simulink model "final_heart_sym4_7_Level_double"  (R2021a)
settings: Solver=VariableStepAuto  StartTime=0.0  StopTime=8  RelTol=1e-3
undefined symbols (not defined in the file): lambda2
libraries: dspsigops x15, dspquant2 x1
(part 2 of 4)

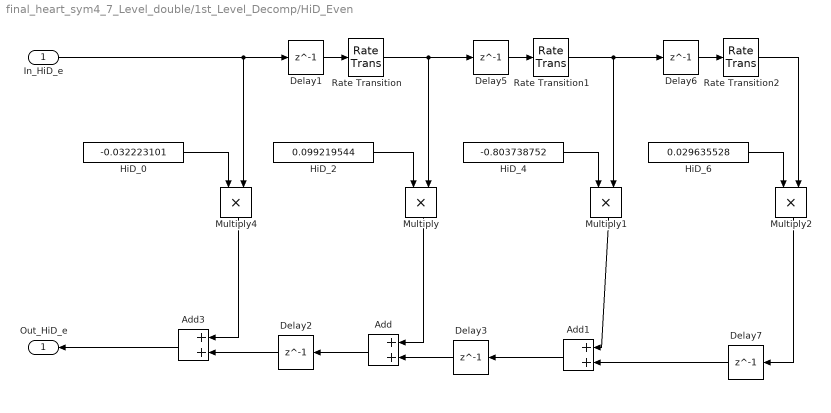
== system final_heart_sym4_7_Level_double/1st_Level_Decomp/HiD_Even ==
  In_HiD_e : Inport  OutDataTypeStr=double  SampleTime=1/44100
  Add : Sum  AccumDataTypeStr=double  OutDataTypeStr=double
  Add1 : Sum  AccumDataTypeStr=double  OutDataTypeStr=double
  Add3 : Sum  AccumDataTypeStr=double  OutDataTypeStr=double
  Delay{1..3,5..7} (6 alike) : Delay  DelayLength=1  SampleTime=1/44100
  HiD_0 : Constant  Value=-0.032223101  OutDataTypeStr=double  SampleTime=1/44100
  HiD_2 : Constant  Value=0.099219544  OutDataTypeStr=double  SampleTime=1/44100
  HiD_4 : Constant  Value=-0.803738752  OutDataTypeStr=double  SampleTime=1/44100
  HiD_6 : Constant  Value=0.029635528  OutDataTypeStr=double  SampleTime=1/44100
  Multiply{,1..2,4} (4 alike) : Product  OutDataTypeStr=double
  Rate Transition : RateTransition  OutPortSampleTime=1/44100
  Rate Transition1 : RateTransition  OutPortSampleTime=1/44100
  Rate Transition2 : RateTransition  OutPortSampleTime=1/44100
  Out_HiD_e : Outport  OutDataTypeStr=double  SampleTime=1/44100  VectorParamsAs1DForOutWhenUnconnected=off
  wires:
  Rate Transition2/1 -> Multiply2/2
  Multiply2/1 -> Delay7/1
  HiD_0/1 -> Multiply4/1
  Delay3/1 -> Add/2
  HiD_6/1 -> Multiply2/1
  In_HiD_e/1 -> Delay1/1, Multiply4/2
  HiD_2/1 -> Multiply/1
  Add3/1 -> Out_HiD_e/1
  Multiply/1 -> Add/1
  Rate Transition/1 -> Delay5/1, Multiply/2
  HiD_4/1 -> Multiply1/1
  Delay6/1 -> Rate Transition2/1
  Delay1/1 -> Rate Transition/1
  Delay7/1 -> Add1/2
  Multiply1/1 -> Add1/1
  Rate Transition1/1 -> Delay6/1, Multiply1/2
  Delay2/1 -> Add3/2
  Multiply4/1 -> Add3/1
  Delay5/1 -> Rate Transition1/1
  Add/1 -> Delay2/1
  Add1/1 -> Delay3/1

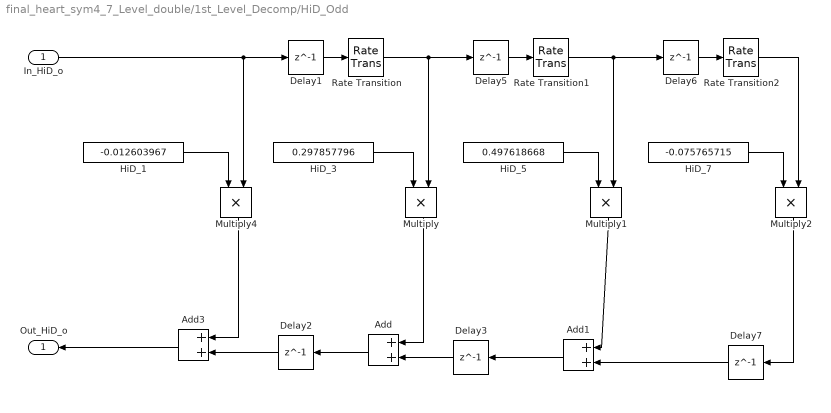
== system final_heart_sym4_7_Level_double/1st_Level_Decomp/HiD_Odd ==
  In_HiD_o : Inport  OutDataTypeStr=double  SampleTime=1/44100
  Add : Sum  AccumDataTypeStr=double  OutDataTypeStr=double
  Add1 : Sum  AccumDataTypeStr=double  OutDataTypeStr=double
  Add3 : Sum  AccumDataTypeStr=double  OutDataTypeStr=double
  Delay{1..3,5..7} (6 alike) : Delay  DelayLength=1  SampleTime=1/44100
  HiD_1 : Constant  Value=-0.012603967  OutDataTypeStr=double  SampleTime=1/44100
  HiD_3 : Constant  Value=0.297857796  OutDataTypeStr=double  SampleTime=1/44100
  HiD_5 : Constant  Value=0.497618668  OutDataTypeStr=double  SampleTime=1/44100
  HiD_7 : Constant  Value=-0.075765715  OutDataTypeStr=double  SampleTime=1/44100
  Multiply{,1..2,4} (4 alike) : Product  OutDataTypeStr=double
  Rate Transition : RateTransition  OutPortSampleTime=1/44100
  Rate Transition1 : RateTransition  OutPortSampleTime=1/44100
  Rate Transition2 : RateTransition  OutPortSampleTime=1/44100
  Out_HiD_o : Outport  OutDataTypeStr=double  SampleTime=1/44100  VectorParamsAs1DForOutWhenUnconnected=off
  wires:
  Delay1/1 -> Rate Transition/1
  Delay6/1 -> Rate Transition2/1
  Rate Transition/1 -> Delay5/1, Multiply/2
  HiD_5/1 -> Multiply1/1
  Rate Transition1/1 -> Delay6/1, Multiply1/2
  Delay2/1 -> Add3/2
  Multiply1/1 -> Add1/1
  Add1/1 -> Delay3/1
  Delay5/1 -> Rate Transition1/1
  Delay7/1 -> Add1/2
  Add/1 -> Delay2/1
  In_HiD_o/1 -> Delay1/1, Multiply4/2
  Multiply4/1 -> Add3/1
  Multiply/1 -> Add/1
  Add3/1 -> Out_HiD_o/1
  HiD_3/1 -> Multiply/1
  HiD_1/1 -> Multiply4/1
  Delay3/1 -> Add/2
  Multiply2/1 -> Delay7/1
  Rate Transition2/1 -> Multiply2/2
  HiD_7/1 -> Multiply2/1

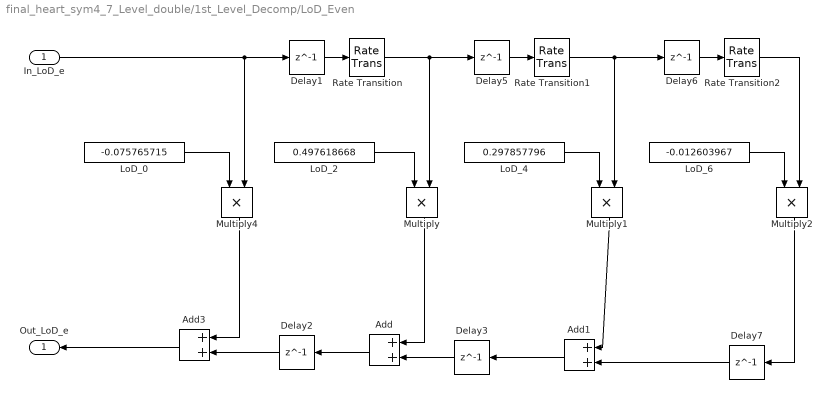
== system final_heart_sym4_7_Level_double/1st_Level_Decomp/LoD_Even ==
  In_LoD_e : Inport  OutDataTypeStr=double  SampleTime=1/44100
  Add : Sum  AccumDataTypeStr=double  OutDataTypeStr=double
  Add1 : Sum  AccumDataTypeStr=double  OutDataTypeStr=double
  Add3 : Sum  AccumDataTypeStr=double  OutDataTypeStr=double
  Delay{1..3,5..7} (6 alike) : Delay  DelayLength=1  SampleTime=1/44100
  LoD_0 : Constant  Value=-0.075765715  OutDataTypeStr=double  SampleTime=1/44100
  LoD_2 : Constant  Value=0.497618668  OutDataTypeStr=double  SampleTime=1/44100
  LoD_4 : Constant  Value=0.297857796  OutDataTypeStr=double  SampleTime=1/44100
  LoD_6 : Constant  Value=-0.012603967  OutDataTypeStr=double  SampleTime=1/44100
  Multiply{,1..2,4} (4 alike) : Product  OutDataTypeStr=double
  Rate Transition : RateTransition  OutPortSampleTime=1/44100
  Rate Transition1 : RateTransition  OutPortSampleTime=1/44100
  Rate Transition2 : RateTransition  OutPortSampleTime=1/44100
  Out_LoD_e : Outport  OutDataTypeStr=double  SampleTime=1/44100  VectorParamsAs1DForOutWhenUnconnected=off
  wires:
  Delay1/1 -> Rate Transition/1
  Delay6/1 -> Rate Transition2/1
  Rate Transition/1 -> Delay5/1, Multiply/2
  LoD_4/1 -> Multiply1/1
  Rate Transition1/1 -> Delay6/1, Multiply1/2
  Delay2/1 -> Add3/2
  Multiply1/1 -> Add1/1
  Add1/1 -> Delay3/1
  Delay5/1 -> Rate Transition1/1
  Delay7/1 -> Add1/2
  Add/1 -> Delay2/1
  In_LoD_e/1 -> Delay1/1, Multiply4/2
  Multiply4/1 -> Add3/1
  Multiply/1 -> Add/1
  Add3/1 -> Out_LoD_e/1
  LoD_2/1 -> Multiply/1
  LoD_0/1 -> Multiply4/1
  Delay3/1 -> Add/2
  Multiply2/1 -> Delay7/1
  Rate Transition2/1 -> Multiply2/2
  LoD_6/1 -> Multiply2/1

== system final_heart_sym4_7_Level_double/1st_Level_Decomp/LoD_Odd ==
  In_LoD_o : Inport  OutDataTypeStr=double  SampleTime=1/44100
  Add : Sum  AccumDataTypeStr=double  OutDataTypeStr=double
  Add1 : Sum  AccumDataTypeStr=double  OutDataTypeStr=double
  Add3 : Sum  AccumDataTypeStr=double  OutDataTypeStr=double
  Delay{1..3,5..7} (6 alike) : Delay  DelayLength=1  SampleTime=1/44100
  LoD_1 : Constant  Value=-0.029635528  OutDataTypeStr=double  SampleTime=1/44100
  LoD_3 : Constant  Value=0.803738752  OutDataTypeStr=double  SampleTime=1/44100
  LoD_5 : Constant  Value=-0.099219544  OutDataTypeStr=double  SampleTime=1/44100
  LoD_7 : Constant  Value=0.032223101  OutDataTypeStr=double  SampleTime=1/44100
  Multiply{,1..2,4} (4 alike) : Product  OutDataTypeStr=double
  Rate Transition : RateTransition  OutPortSampleTime=1/44100
  Rate Transition1 : RateTransition  OutPortSampleTime=1/44100
  Rate Transition2 : RateTransition  OutPortSampleTime=1/44100
  Out_LoD_o : Outport  OutDataTypeStr=double  SampleTime=1/44100  VectorParamsAs1DForOutWhenUnconnected=off
  wires:
  Rate Transition/1 -> Delay5/1, Multiply/2
  Add/1 -> Delay2/1
  Add1/1 -> Delay3/1
  Delay7/1 -> Add1/2
  Delay5/1 -> Rate Transition1/1
  Rate Transition1/1 -> Delay6/1, Multiply1/2
  Delay2/1 -> Add3/2
  LoD_5/1 -> Multiply1/1
  Rate Transition2/1 -> Multiply2/2
  LoD_7/1 -> Multiply2/1
  Multiply2/1 -> Delay7/1
  Delay3/1 -> Add/2
  LoD_3/1 -> Multiply/1
  Add3/1 -> Out_LoD_o/1
  Multiply/1 -> Add/1
  Multiply4/1 -> Add3/1
  Multiply1/1 -> Add1/1
  Delay6/1 -> Rate Transition2/1
  In_LoD_o/1 -> Delay1/1, Multiply4/2
  LoD_1/1 -> Multiply4/1
  Delay1/1 -> Rate Transition/1

== system final_heart_sym4_7_Level_double/1st_Level_Recon/HiR_Even ==
  In_HiR_e : Inport  OutDataTypeStr=double  SampleTime=1/44100
  Add1 : Sum  AccumDataTypeStr=double  OutDataTypeStr=double
  Add2 : Sum  AccumDataTypeStr=double  OutDataTypeStr=double
  Add3 : Sum  AccumDataTypeStr=double  OutDataTypeStr=double
  Delay{1..3,5..7} (6 alike) : Delay  DelayLength=1  SampleTime=1/44100
  HiR_0 : Constant  Value=-0.075765715  OutDataTypeStr=double  SampleTime=1/44100
  HiR_2 : Constant  Value=0.497618668  OutDataTypeStr=double  SampleTime=1/44100
  HiR_4 : Constant  Value=0.297857796  OutDataTypeStr=double  SampleTime=1/44100
  HiR_6 : Constant  Value=-0.012603967  OutDataTypeStr=double  SampleTime=1/44100
  Multiply{1..4} (4 alike) : Product  OutDataTypeStr=double
  Rate Transition : RateTransition  OutPortSampleTime=1/44100
  Rate Transition1 : RateTransition  OutPortSampleTime=1/44100
  Rate Transition2 : RateTransition  OutPortSampleTime=1/44100
  Out_HiR_e : Outport  OutDataTypeStr=double  SampleTime=1/44100  VectorParamsAs1DForOutWhenUnconnected=off
  wires:
  In_HiR_e/1 -> Delay1/1, Multiply4/2
  Delay6/1 -> Rate Transition2/1
  Multiply2/1 -> Add2/1
  Rate Transition/1 -> Delay5/1, Multiply1/2
  HiR_6/1 -> Multiply3/1
  Multiply3/1 -> Delay2/1
  Delay2/1 -> Add2/2
  Rate Transition2/1 -> Multiply3/2
  Add3/1 -> Out_HiR_e/1
  Multiply1/1 -> Add1/1
  Delay1/1 -> Rate Transition/1
  Multiply4/1 -> Add3/1
  Add1/1 -> Delay7/1
  Add2/1 -> Delay3/1
  HiR_2/1 -> Multiply1/1
  HiR_4/1 -> Multiply2/1
  Delay7/1 -> Add3/2
  HiR_0/1 -> Multiply4/1
  Delay3/1 -> Add1/2
  Delay5/1 -> Rate Transition1/1
  Rate Transition1/1 -> Delay6/1, Multiply2/2

== system final_heart_sym4_7_Level_double/1st_Level_Recon/HiR_Odd ==
  In_HiR_o : Inport  OutDataTypeStr=double  SampleTime=1/44100
  Add1 : Sum  AccumDataTypeStr=double  OutDataTypeStr=double
  Add2 : Sum  AccumDataTypeStr=double  OutDataTypeStr=double
  Add3 : Sum  AccumDataTypeStr=double  OutDataTypeStr=double
  Delay{1..3,5..7} (6 alike) : Delay  DelayLength=1  SampleTime=1/44100
  HiR_1 : Constant  Value=0.029635528  OutDataTypeStr=double  SampleTime=1/44100
  HiR_3 : Constant  Value=-0.803738752  OutDataTypeStr=double  SampleTime=1/44100
  HiR_5 : Constant  Value=0.099219544  OutDataTypeStr=double  SampleTime=1/44100
  HiR_7 : Constant  Value=-0.032223101  OutDataTypeStr=double  SampleTime=1/44100
  Multiply{1..4} (4 alike) : Product  OutDataTypeStr=double
  Rate Transition : RateTransition  OutPortSampleTime=1/44100
  Rate Transition1 : RateTransition  OutPortSampleTime=1/44100
  Rate Transition2 : RateTransition  OutPortSampleTime=1/44100
  Out_HiR_o : Outport  OutDataTypeStr=double  SampleTime=1/44100  VectorParamsAs1DForOutWhenUnconnected=off
  wires:
  Delay1/1 -> Rate Transition/1
  Multiply1/1 -> Add1/1
  Multiply3/1 -> Delay2/1
  Rate Transition2/1 -> Multiply3/2
  Delay2/1 -> Add2/2
  Rate Transition/1 -> Delay5/1, Multiply1/2
  Multiply2/1 -> Add2/1
  Add3/1 -> Out_HiR_o/1
  Delay6/1 -> Rate Transition2/1
  In_HiR_o/1 -> Delay1/1, Multiply4/2
  Delay7/1 -> Add3/2
  Multiply4/1 -> Add3/1
  HiR_3/1 -> Multiply1/1
  Add2/1 -> Delay3/1
  Delay5/1 -> Rate Transition1/1
  HiR_5/1 -> Multiply2/1
  Delay3/1 -> Add1/2
  Rate Transition1/1 -> Delay6/1, Multiply2/2
  Add1/1 -> Delay7/1
  HiR_1/1 -> Multiply4/1
  HiR_7/1 -> Multiply3/1

== system final_heart_sym4_7_Level_double/1st_Level_Recon/LoR_Even ==
  In_LoR_e : Inport  OutDataTypeStr=double  SampleTime=1/44100
  Add1 : Sum  AccumDataTypeStr=double  OutDataTypeStr=double
  Add2 : Sum  AccumDataTypeStr=double  OutDataTypeStr=double
  Add3 : Sum  AccumDataTypeStr=double  OutDataTypeStr=double
  Delay{1..3,5..7} (6 alike) : Delay  DelayLength=1  SampleTime=1/44100
  LoR_0 : Constant  Value=0.032223101  OutDataTypeStr=double  SampleTime=1/44100
  LoR_2 : Constant  Value=-0.099219544  OutDataTypeStr=double  SampleTime=1/44100
  LoR_4 : Constant  Value=0.803738752  OutDataTypeStr=double  SampleTime=1/44100
  LoR_6 : Constant  Value=-0.029635528  OutDataTypeStr=double  SampleTime=1/44100
  Multiply{1..4} (4 alike) : Product  OutDataTypeStr=double
  Rate Transition : RateTransition  OutPortSampleTime=1/44100
  Rate Transition1 : RateTransition  OutPortSampleTime=1/44100
  Rate Transition2 : RateTransition  OutPortSampleTime=1/44100
  Out_LoR_e : Outport  OutDataTypeStr=double  SampleTime=1/44100  VectorParamsAs1DForOutWhenUnconnected=off
  wires:
  Delay1/1 -> Rate Transition/1
  Multiply1/1 -> Add1/1
  Multiply3/1 -> Delay2/1
  Rate Transition2/1 -> Multiply3/2
  Delay2/1 -> Add2/2
  Rate Transition/1 -> Delay5/1, Multiply1/2
  Multiply2/1 -> Add2/1
  Add3/1 -> Out_LoR_e/1
  Delay6/1 -> Rate Transition2/1
  In_LoR_e/1 -> Delay1/1, Multiply4/2
  Delay7/1 -> Add3/2
  Multiply4/1 -> Add3/1
  LoR_2/1 -> Multiply1/1
  Add2/1 -> Delay3/1
  Delay5/1 -> Rate Transition1/1
  LoR_4/1 -> Multiply2/1
  Delay3/1 -> Add1/2
  Rate Transition1/1 -> Delay6/1, Multiply2/2
  Add1/1 -> Delay7/1
  LoR_0/1 -> Multiply4/1
  LoR_6/1 -> Multiply3/1

== system final_heart_sym4_7_Level_double/1st_Level_Recon/LoR_Odd ==
  In_LoR_o : Inport  OutDataTypeStr=double  SampleTime=1/44100
  Add1 : Sum  AccumDataTypeStr=double  OutDataTypeStr=double
  Add2 : Sum  AccumDataTypeStr=double  OutDataTypeStr=double
  Add3 : Sum  AccumDataTypeStr=double  OutDataTypeStr=double
  Delay{1..3,5..7} (6 alike) : Delay  DelayLength=1  SampleTime=1/44100
  LoR_1 : Constant  Value=-0.012603967  OutDataTypeStr=double  SampleTime=1/44100
  LoR_3 : Constant  Value=0.297857796  OutDataTypeStr=double  SampleTime=1/44100
  LoR_5 : Constant  Value=0.497618668  OutDataTypeStr=double  SampleTime=1/44100
  LoR_7 : Constant  Value=-0.075765715  OutDataTypeStr=double  SampleTime=1/44100
  Multiply{1..4} (4 alike) : Product  OutDataTypeStr=double
  Rate Transition : RateTransition  OutPortSampleTime=1/44100
  Rate Transition1 : RateTransition  OutPortSampleTime=1/44100
  Rate Transition2 : RateTransition  OutPortSampleTime=1/44100
  Out_LoR_o : Outport  OutDataTypeStr=double  SampleTime=1/44100  VectorParamsAs1DForOutWhenUnconnected=off
  wires:
  Rate Transition1/1 -> Delay6/1, Multiply2/2
  Add1/1 -> Delay7/1
  LoR_1/1 -> Multiply4/1
  LoR_7/1 -> Multiply3/1
  Delay3/1 -> Add1/2
  LoR_3/1 -> Multiply1/1
  Add2/1 -> Delay3/1
  LoR_5/1 -> Multiply2/1
  Delay5/1 -> Rate Transition1/1
  In_LoR_o/1 -> Delay1/1, Multiply4/2
  Multiply4/1 -> Add3/1
  Delay7/1 -> Add3/2
  Multiply2/1 -> Add2/1
  Rate Transition/1 -> Delay5/1, Multiply1/2
  Delay6/1 -> Rate Transition2/1
  Add3/1 -> Out_LoR_o/1
  Delay2/1 -> Add2/2
  Multiply3/1 -> Delay2/1
  Rate Transition2/1 -> Multiply3/2
  Multiply1/1 -> Add1/1
  Delay1/1 -> Rate Transition/1

== system final_heart_sym4_7_Level_double/2nd_Level_Decomp/HiD_Even ==
  In_HiD_e : Inport  OutDataTypeStr=double  SampleTime=1/44100
  Add : Sum  AccumDataTypeStr=double  OutDataTypeStr=double
  Add1 : Sum  AccumDataTypeStr=double  OutDataTypeStr=double
  Add3 : Sum  AccumDataTypeStr=double  OutDataTypeStr=double
  Delay{1..3,5..7} (6 alike) : Delay  DelayLength=1  SampleTime=1/44100
  HiD_0 : Constant  Value=-0.032223101  OutDataTypeStr=double  SampleTime=1/44100
  HiD_2 : Constant  Value=0.099219544  OutDataTypeStr=double  SampleTime=1/44100
  HiD_4 : Constant  Value=-0.803738752  OutDataTypeStr=double  SampleTime=1/44100
  HiD_6 : Constant  Value=0.029635528  OutDataTypeStr=double  SampleTime=1/44100
  Multiply{,1..2,4} (4 alike) : Product  OutDataTypeStr=double
  Rate Transition : RateTransition  OutPortSampleTime=1/44100
  Rate Transition1 : RateTransition  OutPortSampleTime=1/44100
  Rate Transition2 : RateTransition  OutPortSampleTime=1/44100
  Out_HiD_e : Outport  OutDataTypeStr=double  SampleTime=1/44100  VectorParamsAs1DForOutWhenUnconnected=off
  wires:
  Rate Transition2/1 -> Multiply2/2
  Multiply2/1 -> Delay7/1
  HiD_0/1 -> Multiply4/1
  Delay3/1 -> Add/2
  HiD_6/1 -> Multiply2/1
  In_HiD_e/1 -> Delay1/1, Multiply4/2
  HiD_2/1 -> Multiply/1
  Add3/1 -> Out_HiD_e/1
  Multiply/1 -> Add/1
  Rate Transition/1 -> Delay5/1, Multiply/2
  HiD_4/1 -> Multiply1/1
  Delay6/1 -> Rate Transition2/1
  Delay1/1 -> Rate Transition/1
  Delay7/1 -> Add1/2
  Multiply1/1 -> Add1/1
  Rate Transition1/1 -> Delay6/1, Multiply1/2
  Delay2/1 -> Add3/2
  Multiply4/1 -> Add3/1
  Delay5/1 -> Rate Transition1/1
  Add/1 -> Delay2/1
  Add1/1 -> Delay3/1

== system final_heart_sym4_7_Level_double/2nd_Level_Decomp/HiD_Odd ==
  In_HiD_o : Inport  OutDataTypeStr=double  SampleTime=1/44100
  Add : Sum  AccumDataTypeStr=double  OutDataTypeStr=double
  Add1 : Sum  AccumDataTypeStr=double  OutDataTypeStr=double
  Add3 : Sum  AccumDataTypeStr=double  OutDataTypeStr=double
  Delay{1..3,5..7} (6 alike) : Delay  DelayLength=1  SampleTime=1/44100
  HiD_1 : Constant  Value=-0.012603967  OutDataTypeStr=double  SampleTime=1/44100
  HiD_3 : Constant  Value=0.297857796  OutDataTypeStr=double  SampleTime=1/44100
  HiD_5 : Constant  Value=0.497618668  OutDataTypeStr=double  SampleTime=1/44100
  HiD_7 : Constant  Value=-0.075765715  OutDataTypeStr=double  SampleTime=1/44100
  Multiply{,1..2,4} (4 alike) : Product  OutDataTypeStr=double
  Rate Transition : RateTransition  OutPortSampleTime=1/44100
  Rate Transition1 : RateTransition  OutPortSampleTime=1/44100
  Rate Transition2 : RateTransition  OutPortSampleTime=1/44100
  Out_HiD_o : Outport  OutDataTypeStr=double  SampleTime=1/44100  VectorParamsAs1DForOutWhenUnconnected=off
  wires:
  Delay1/1 -> Rate Transition/1
  Delay6/1 -> Rate Transition2/1
  Rate Transition/1 -> Delay5/1, Multiply/2
  HiD_5/1 -> Multiply1/1
  Rate Transition1/1 -> Delay6/1, Multiply1/2
  Delay2/1 -> Add3/2
  Multiply1/1 -> Add1/1
  Add1/1 -> Delay3/1
  Delay5/1 -> Rate Transition1/1
  Delay7/1 -> Add1/2
  Add/1 -> Delay2/1
  In_HiD_o/1 -> Delay1/1, Multiply4/2
  Multiply4/1 -> Add3/1
  Multiply/1 -> Add/1
  Add3/1 -> Out_HiD_o/1
  HiD_3/1 -> Multiply/1
  HiD_1/1 -> Multiply4/1
  Delay3/1 -> Add/2
  Multiply2/1 -> Delay7/1
  Rate Transition2/1 -> Multiply2/2
  HiD_7/1 -> Multiply2/1

== system final_heart_sym4_7_Level_double/2nd_Level_Decomp/LoD_Even ==
  In_LoD_e : Inport  OutDataTypeStr=double  SampleTime=1/44100
  Add : Sum  AccumDataTypeStr=double  OutDataTypeStr=double
  Add1 : Sum  AccumDataTypeStr=double  OutDataTypeStr=double
  Add3 : Sum  AccumDataTypeStr=double  OutDataTypeStr=double
  Delay{1..3,5..7} (6 alike) : Delay  DelayLength=1  SampleTime=1/44100
  LoD_0 : Constant  Value=-0.075765715  OutDataTypeStr=double  SampleTime=1/44100
  LoD_2 : Constant  Value=0.497618668  OutDataTypeStr=double  SampleTime=1/44100
  LoD_4 : Constant  Value=0.297857796  OutDataTypeStr=double  SampleTime=1/44100
  LoD_6 : Constant  Value=-0.012603967  OutDataTypeStr=double  SampleTime=1/44100
  Multiply{,1..2,4} (4 alike) : Product  OutDataTypeStr=double
  Rate Transition : RateTransition  OutPortSampleTime=1/44100
  Rate Transition1 : RateTransition  OutPortSampleTime=1/44100
  Rate Transition2 : RateTransition  OutPortSampleTime=1/44100
  Out_LoD_e : Outport  OutDataTypeStr=double  SampleTime=1/44100  VectorParamsAs1DForOutWhenUnconnected=off
  wires:
  Delay1/1 -> Rate Transition/1
  Delay6/1 -> Rate Transition2/1
  Rate Transition/1 -> Delay5/1, Multiply/2
  LoD_4/1 -> Multiply1/1
  Rate Transition1/1 -> Delay6/1, Multiply1/2
  Delay2/1 -> Add3/2
  Multiply1/1 -> Add1/1
  Add1/1 -> Delay3/1
  Delay5/1 -> Rate Transition1/1
  Delay7/1 -> Add1/2
  Add/1 -> Delay2/1
  In_LoD_e/1 -> Delay1/1, Multiply4/2
  Multiply4/1 -> Add3/1
  Multiply/1 -> Add/1
  Add3/1 -> Out_LoD_e/1
  LoD_2/1 -> Multiply/1
  LoD_0/1 -> Multiply4/1
  Delay3/1 -> Add/2
  Multiply2/1 -> Delay7/1
  Rate Transition2/1 -> Multiply2/2
  LoD_6/1 -> Multiply2/1

== system final_heart_sym4_7_Level_double/2nd_Level_Decomp/LoD_Odd ==
  In_LoD_o : Inport  OutDataTypeStr=double  SampleTime=1/44100
  Add : Sum  AccumDataTypeStr=double  OutDataTypeStr=double
  Add1 : Sum  AccumDataTypeStr=double  OutDataTypeStr=double
  Add3 : Sum  AccumDataTypeStr=double  OutDataTypeStr=double
  Delay{1..3,5..7} (6 alike) : Delay  DelayLength=1  SampleTime=1/44100
  LoD_1 : Constant  Value=-0.029635528  OutDataTypeStr=double  SampleTime=1/44100
  LoD_3 : Constant  Value=0.803738752  OutDataTypeStr=double  SampleTime=1/44100
  LoD_5 : Constant  Value=-0.099219544  OutDataTypeStr=double  SampleTime=1/44100
  LoD_7 : Constant  Value=0.032223101  OutDataTypeStr=double  SampleTime=1/44100
  Multiply{,1..2,4} (4 alike) : Product  OutDataTypeStr=double
  Rate Transition : RateTransition  OutPortSampleTime=1/44100
  Rate Transition1 : RateTransition  OutPortSampleTime=1/44100
  Rate Transition2 : RateTransition  OutPortSampleTime=1/44100
  Out_LoD_o : Outport  OutDataTypeStr=double  SampleTime=1/44100  VectorParamsAs1DForOutWhenUnconnected=off
  wires:
  Rate Transition/1 -> Delay5/1, Multiply/2
  Add/1 -> Delay2/1
  Add1/1 -> Delay3/1
  Delay7/1 -> Add1/2
  Delay5/1 -> Rate Transition1/1
  Rate Transition1/1 -> Delay6/1, Multiply1/2
  Delay2/1 -> Add3/2
  LoD_5/1 -> Multiply1/1
  Rate Transition2/1 -> Multiply2/2
  LoD_7/1 -> Multiply2/1
  Multiply2/1 -> Delay7/1
  Delay3/1 -> Add/2
  LoD_3/1 -> Multiply/1
  Add3/1 -> Out_LoD_o/1
  Multiply/1 -> Add/1
  Multiply4/1 -> Add3/1
  Multiply1/1 -> Add1/1
  Delay6/1 -> Rate Transition2/1
  In_LoD_o/1 -> Delay1/1, Multiply4/2
  LoD_1/1 -> Multiply4/1
  Delay1/1 -> Rate Transition/1

== system final_heart_sym4_7_Level_double/2nd_Level_Recon/HiR_Even ==
  In_HiR_e : Inport  OutDataTypeStr=double  SampleTime=1/44100
  Add1 : Sum  AccumDataTypeStr=double  OutDataTypeStr=double
  Add2 : Sum  AccumDataTypeStr=double  OutDataTypeStr=double
  Add3 : Sum  AccumDataTypeStr=double  OutDataTypeStr=double
  Delay{1..3,5..7} (6 alike) : Delay  DelayLength=1  SampleTime=1/44100
  HiR_0 : Constant  Value=-0.075765715  OutDataTypeStr=double  SampleTime=1/44100
  HiR_2 : Constant  Value=0.497618668  OutDataTypeStr=double  SampleTime=1/44100
  HiR_4 : Constant  Value=0.297857796  OutDataTypeStr=double  SampleTime=1/44100
  HiR_6 : Constant  Value=-0.012603967  OutDataTypeStr=double  SampleTime=1/44100
  Multiply{1..4} (4 alike) : Product  OutDataTypeStr=double
  Rate Transition : RateTransition  OutPortSampleTime=1/44100
  Rate Transition1 : RateTransition  OutPortSampleTime=1/44100
  Rate Transition2 : RateTransition  OutPortSampleTime=1/44100
  Out_HiR_e : Outport  OutDataTypeStr=double  SampleTime=1/44100  VectorParamsAs1DForOutWhenUnconnected=off
  wires:
  In_HiR_e/1 -> Delay1/1, Multiply4/2
  Delay6/1 -> Rate Transition2/1
  Multiply2/1 -> Add2/1
  Rate Transition/1 -> Delay5/1, Multiply1/2
  HiR_6/1 -> Multiply3/1
  Multiply3/1 -> Delay2/1
  Delay2/1 -> Add2/2
  Rate Transition2/1 -> Multiply3/2
  Add3/1 -> Out_HiR_e/1
  Multiply1/1 -> Add1/1
  Delay1/1 -> Rate Transition/1
  Multiply4/1 -> Add3/1
  Add1/1 -> Delay7/1
  Add2/1 -> Delay3/1
  HiR_2/1 -> Multiply1/1
  HiR_4/1 -> Multiply2/1
  Delay7/1 -> Add3/2
  HiR_0/1 -> Multiply4/1
  Delay3/1 -> Add1/2
  Delay5/1 -> Rate Transition1/1
  Rate Transition1/1 -> Delay6/1, Multiply2/2

== system final_heart_sym4_7_Level_double/2nd_Level_Recon/HiR_Odd ==
  In_HiR_o : Inport  OutDataTypeStr=double  SampleTime=1/44100
  Add1 : Sum  AccumDataTypeStr=double  OutDataTypeStr=double
  Add2 : Sum  AccumDataTypeStr=double  OutDataTypeStr=double
  Add3 : Sum  AccumDataTypeStr=double  OutDataTypeStr=double
  Delay{1..3,5..7} (6 alike) : Delay  DelayLength=1  SampleTime=1/44100
  HiR_1 : Constant  Value=0.029635528  OutDataTypeStr=double  SampleTime=1/44100
  HiR_3 : Constant  Value=-0.803738752  OutDataTypeStr=double  SampleTime=1/44100
  HiR_5 : Constant  Value=0.099219544  OutDataTypeStr=double  SampleTime=1/44100
  HiR_7 : Constant  Value=-0.032223101  OutDataTypeStr=double  SampleTime=1/44100
  Multiply{1..4} (4 alike) : Product  OutDataTypeStr=double
  Rate Transition : RateTransition  OutPortSampleTime=1/44100
  Rate Transition1 : RateTransition  OutPortSampleTime=1/44100
  Rate Transition2 : RateTransition  OutPortSampleTime=1/44100
  Out_HiR_o : Outport  OutDataTypeStr=double  SampleTime=1/44100  VectorParamsAs1DForOutWhenUnconnected=off
  wires:
  Delay1/1 -> Rate Transition/1
  Multiply1/1 -> Add1/1
  Multiply3/1 -> Delay2/1
  Rate Transition2/1 -> Multiply3/2
  Delay2/1 -> Add2/2
  Rate Transition/1 -> Delay5/1, Multiply1/2
  Multiply2/1 -> Add2/1
  Add3/1 -> Out_HiR_o/1
  Delay6/1 -> Rate Transition2/1
  In_HiR_o/1 -> Delay1/1, Multiply4/2
  Delay7/1 -> Add3/2
  Multiply4/1 -> Add3/1
  HiR_3/1 -> Multiply1/1
  Add2/1 -> Delay3/1
  Delay5/1 -> Rate Transition1/1
  HiR_5/1 -> Multiply2/1
  Delay3/1 -> Add1/2
  Rate Transition1/1 -> Delay6/1, Multiply2/2
  Add1/1 -> Delay7/1
  HiR_1/1 -> Multiply4/1
  HiR_7/1 -> Multiply3/1

== system final_heart_sym4_7_Level_double/2nd_Level_Recon/LoR_Even ==
  In_LoR_e : Inport  OutDataTypeStr=double  SampleTime=1/44100
  Add1 : Sum  AccumDataTypeStr=double  OutDataTypeStr=double
  Add2 : Sum  AccumDataTypeStr=double  OutDataTypeStr=double
  Add3 : Sum  AccumDataTypeStr=double  OutDataTypeStr=double
  Delay{1..3,5..7} (6 alike) : Delay  DelayLength=1  SampleTime=1/44100
  LoR_0 : Constant  Value=0.032223101  OutDataTypeStr=double  SampleTime=1/44100
  LoR_2 : Constant  Value=-0.099219544  OutDataTypeStr=double  SampleTime=1/44100
  LoR_4 : Constant  Value=0.803738752  OutDataTypeStr=double  SampleTime=1/44100
  LoR_6 : Constant  Value=-0.029635528  OutDataTypeStr=double  SampleTime=1/44100
  Multiply{1..4} (4 alike) : Product  OutDataTypeStr=double
  Rate Transition : RateTransition  OutPortSampleTime=1/44100
  Rate Transition1 : RateTransition  OutPortSampleTime=1/44100
  Rate Transition2 : RateTransition  OutPortSampleTime=1/44100
  Out_LoR_e : Outport  OutDataTypeStr=double  SampleTime=1/44100  VectorParamsAs1DForOutWhenUnconnected=off
  wires:
  Delay1/1 -> Rate Transition/1
  Multiply1/1 -> Add1/1
  Multiply3/1 -> Delay2/1
  Rate Transition2/1 -> Multiply3/2
  Delay2/1 -> Add2/2
  Rate Transition/1 -> Delay5/1, Multiply1/2
  Multiply2/1 -> Add2/1
  Add3/1 -> Out_LoR_e/1
  Delay6/1 -> Rate Transition2/1
  In_LoR_e/1 -> Delay1/1, Multiply4/2
  Delay7/1 -> Add3/2
  Multiply4/1 -> Add3/1
  LoR_2/1 -> Multiply1/1
  Add2/1 -> Delay3/1
  Delay5/1 -> Rate Transition1/1
  LoR_4/1 -> Multiply2/1
  Delay3/1 -> Add1/2
  Rate Transition1/1 -> Delay6/1, Multiply2/2
  Add1/1 -> Delay7/1
  LoR_0/1 -> Multiply4/1
  LoR_6/1 -> Multiply3/1

== system final_heart_sym4_7_Level_double/2nd_Level_Recon/LoR_Odd ==
  In_LoR_o : Inport  OutDataTypeStr=double  SampleTime=1/44100
  Add1 : Sum  AccumDataTypeStr=double  OutDataTypeStr=double
  Add2 : Sum  AccumDataTypeStr=double  OutDataTypeStr=double
  Add3 : Sum  AccumDataTypeStr=double  OutDataTypeStr=double
  Delay{1..3,5..7} (6 alike) : Delay  DelayLength=1  SampleTime=1/44100
  LoR_1 : Constant  Value=-0.012603967  OutDataTypeStr=double  SampleTime=1/44100
  LoR_3 : Constant  Value=0.297857796  OutDataTypeStr=double  SampleTime=1/44100
  LoR_5 : Constant  Value=0.497618668  OutDataTypeStr=double  SampleTime=1/44100
  LoR_7 : Constant  Value=-0.075765715  OutDataTypeStr=double  SampleTime=1/44100
  Multiply{1..4} (4 alike) : Product  OutDataTypeStr=double
  Rate Transition : RateTransition  OutPortSampleTime=1/44100
  Rate Transition1 : RateTransition  OutPortSampleTime=1/44100
  Rate Transition2 : RateTransition  OutPortSampleTime=1/44100
  Out_LoR_o : Outport  OutDataTypeStr=double  SampleTime=1/44100  VectorParamsAs1DForOutWhenUnconnected=off
  wires:
  Rate Transition1/1 -> Delay6/1, Multiply2/2
  Add1/1 -> Delay7/1
  LoR_1/1 -> Multiply4/1
  LoR_7/1 -> Multiply3/1
  Delay3/1 -> Add1/2
  LoR_3/1 -> Multiply1/1
  Add2/1 -> Delay3/1
  LoR_5/1 -> Multiply2/1
  Delay5/1 -> Rate Transition1/1
  In_LoR_o/1 -> Delay1/1, Multiply4/2
  Multiply4/1 -> Add3/1
  Delay7/1 -> Add3/2
  Multiply2/1 -> Add2/1
  Rate Transition/1 -> Delay5/1, Multiply1/2
  Delay6/1 -> Rate Transition2/1
  Add3/1 -> Out_LoR_o/1
  Delay2/1 -> Add2/2
  Multiply3/1 -> Delay2/1
  Rate Transition2/1 -> Multiply3/2
  Multiply1/1 -> Add1/1
  Delay1/1 -> Rate Transition/1

== system final_heart_sym4_7_Level_double/3rd_Level_Decomp/HiD_Even ==
  In_HiD_e : Inport  OutDataTypeStr=double  SampleTime=1/44100
  Add : Sum  AccumDataTypeStr=double  OutDataTypeStr=double
  Add1 : Sum  AccumDataTypeStr=double  OutDataTypeStr=double
  Add3 : Sum  AccumDataTypeStr=double  OutDataTypeStr=double
  Delay{1..3,5..7} (6 alike) : Delay  DelayLength=1  SampleTime=1/44100
  HiD_0 : Constant  Value=-0.032223101  OutDataTypeStr=double  SampleTime=1/44100
  HiD_2 : Constant  Value=0.099219544  OutDataTypeStr=double  SampleTime=1/44100
  HiD_4 : Constant  Value=-0.803738752  OutDataTypeStr=double  SampleTime=1/44100
  HiD_6 : Constant  Value=0.029635528  OutDataTypeStr=double  SampleTime=1/44100
  Multiply{,1..2,4} (4 alike) : Product  OutDataTypeStr=double
  Rate Transition : RateTransition  OutPortSampleTime=1/44100
  Rate Transition1 : RateTransition  OutPortSampleTime=1/44100
  Rate Transition2 : RateTransition  OutPortSampleTime=1/44100
  Out_HiD_e : Outport  OutDataTypeStr=double  SampleTime=1/44100  VectorParamsAs1DForOutWhenUnconnected=off
  wires:
  Rate Transition2/1 -> Multiply2/2
  Multiply2/1 -> Delay7/1
  HiD_0/1 -> Multiply4/1
  Delay3/1 -> Add/2
  HiD_6/1 -> Multiply2/1
  In_HiD_e/1 -> Delay1/1, Multiply4/2
  HiD_2/1 -> Multiply/1
  Add3/1 -> Out_HiD_e/1
  Multiply/1 -> Add/1
  Rate Transition/1 -> Delay5/1, Multiply/2
  HiD_4/1 -> Multiply1/1
  Delay6/1 -> Rate Transition2/1
  Delay1/1 -> Rate Transition/1
  Delay7/1 -> Add1/2
  Multiply1/1 -> Add1/1
  Rate Transition1/1 -> Delay6/1, Multiply1/2
  Delay2/1 -> Add3/2
  Multiply4/1 -> Add3/1
  Delay5/1 -> Rate Transition1/1
  Add/1 -> Delay2/1
  Add1/1 -> Delay3/1

== system final_heart_sym4_7_Level_double/3rd_Level_Decomp/HiD_Odd ==
  In_HiD_o : Inport  OutDataTypeStr=double  SampleTime=1/44100
  Add : Sum  AccumDataTypeStr=double  OutDataTypeStr=double
  Add1 : Sum  AccumDataTypeStr=double  OutDataTypeStr=double
  Add3 : Sum  AccumDataTypeStr=double  OutDataTypeStr=double
  Delay{1..3,5..7} (6 alike) : Delay  DelayLength=1  SampleTime=1/44100
  HiD_1 : Constant  Value=-0.012603967  OutDataTypeStr=double  SampleTime=1/44100
  HiD_3 : Constant  Value=0.297857796  OutDataTypeStr=double  SampleTime=1/44100
  HiD_5 : Constant  Value=0.497618668  OutDataTypeStr=double  SampleTime=1/44100
  HiD_7 : Constant  Value=-0.075765715  OutDataTypeStr=double  SampleTime=1/44100
  Multiply{,1..2,4} (4 alike) : Product  OutDataTypeStr=double
  Rate Transition : RateTransition  OutPortSampleTime=1/44100
  Rate Transition1 : RateTransition  OutPortSampleTime=1/44100
  Rate Transition2 : RateTransition  OutPortSampleTime=1/44100
  Out_HiD_o : Outport  OutDataTypeStr=double  SampleTime=1/44100  VectorParamsAs1DForOutWhenUnconnected=off
  wires:
  Delay1/1 -> Rate Transition/1
  Delay6/1 -> Rate Transition2/1
  Rate Transition/1 -> Delay5/1, Multiply/2
  HiD_5/1 -> Multiply1/1
  Rate Transition1/1 -> Delay6/1, Multiply1/2
  Delay2/1 -> Add3/2
  Multiply1/1 -> Add1/1
  Add1/1 -> Delay3/1
  Delay5/1 -> Rate Transition1/1
  Delay7/1 -> Add1/2
  Add/1 -> Delay2/1
  In_HiD_o/1 -> Delay1/1, Multiply4/2
  Multiply4/1 -> Add3/1
  Multiply/1 -> Add/1
  Add3/1 -> Out_HiD_o/1
  HiD_3/1 -> Multiply/1
  HiD_1/1 -> Multiply4/1
  Delay3/1 -> Add/2
  Multiply2/1 -> Delay7/1
  Rate Transition2/1 -> Multiply2/2
  HiD_7/1 -> Multiply2/1

== system final_heart_sym4_7_Level_double/3rd_Level_Decomp/LoD_Even ==
  In_LoD_e : Inport  OutDataTypeStr=double  SampleTime=1/44100
  Add : Sum  AccumDataTypeStr=double  OutDataTypeStr=double
  Add1 : Sum  AccumDataTypeStr=double  OutDataTypeStr=double
  Add3 : Sum  AccumDataTypeStr=double  OutDataTypeStr=double
  Delay{1..3,5..7} (6 alike) : Delay  DelayLength=1  SampleTime=1/44100
  LoD_0 : Constant  Value=-0.075765715  OutDataTypeStr=double  SampleTime=1/44100
  LoD_2 : Constant  Value=0.497618668  OutDataTypeStr=double  SampleTime=1/44100
  LoD_4 : Constant  Value=0.297857796  OutDataTypeStr=double  SampleTime=1/44100
  LoD_6 : Constant  Value=-0.012603967  OutDataTypeStr=double  SampleTime=1/44100
  Multiply{,1..2,4} (4 alike) : Product  OutDataTypeStr=double
  Rate Transition : RateTransition  OutPortSampleTime=1/44100
  Rate Transition1 : RateTransition  OutPortSampleTime=1/44100
  Rate Transition2 : RateTransition  OutPortSampleTime=1/44100
  Out_LoD_e : Outport  OutDataTypeStr=double  SampleTime=1/44100  VectorParamsAs1DForOutWhenUnconnected=off
  wires:
  Delay1/1 -> Rate Transition/1
  Delay6/1 -> Rate Transition2/1
  Rate Transition/1 -> Delay5/1, Multiply/2
  LoD_4/1 -> Multiply1/1
  Rate Transition1/1 -> Delay6/1, Multiply1/2
  Delay2/1 -> Add3/2
  Multiply1/1 -> Add1/1
  Add1/1 -> Delay3/1
  Delay5/1 -> Rate Transition1/1
  Delay7/1 -> Add1/2
  Add/1 -> Delay2/1
  In_LoD_e/1 -> Delay1/1, Multiply4/2
  Multiply4/1 -> Add3/1
  Multiply/1 -> Add/1
  Add3/1 -> Out_LoD_e/1
  LoD_2/1 -> Multiply/1
  LoD_0/1 -> Multiply4/1
  Delay3/1 -> Add/2
  Multiply2/1 -> Delay7/1
  Rate Transition2/1 -> Multiply2/2
  LoD_6/1 -> Multiply2/1

== system final_heart_sym4_7_Level_double/3rd_Level_Decomp/LoD_Odd ==
  In_LoD_o : Inport  OutDataTypeStr=double  SampleTime=1/44100
  Add : Sum  AccumDataTypeStr=double  OutDataTypeStr=double
  Add1 : Sum  AccumDataTypeStr=double  OutDataTypeStr=double
  Add3 : Sum  AccumDataTypeStr=double  OutDataTypeStr=double
  Delay{1..3,5..7} (6 alike) : Delay  DelayLength=1  SampleTime=1/44100
  LoD_1 : Constant  Value=-0.029635528  OutDataTypeStr=double  SampleTime=1/44100
  LoD_3 : Constant  Value=0.803738752  OutDataTypeStr=double  SampleTime=1/44100
  LoD_5 : Constant  Value=-0.099219544  OutDataTypeStr=double  SampleTime=1/44100
  LoD_7 : Constant  Value=0.032223101  OutDataTypeStr=double  SampleTime=1/44100
  Multiply{,1..2,4} (4 alike) : Product  OutDataTypeStr=double
  Rate Transition : RateTransition  OutPortSampleTime=1/44100
  Rate Transition1 : RateTransition  OutPortSampleTime=1/44100
  Rate Transition2 : RateTransition  OutPortSampleTime=1/44100
  Out_LoD_o : Outport  OutDataTypeStr=double  SampleTime=1/44100  VectorParamsAs1DForOutWhenUnconnected=off
  wires:
  Rate Transition/1 -> Delay5/1, Multiply/2
  Add/1 -> Delay2/1
  Add1/1 -> Delay3/1
  Delay7/1 -> Add1/2
  Delay5/1 -> Rate Transition1/1
  Rate Transition1/1 -> Delay6/1, Multiply1/2
  Delay2/1 -> Add3/2
  LoD_5/1 -> Multiply1/1
  Rate Transition2/1 -> Multiply2/2
  LoD_7/1 -> Multiply2/1
  Multiply2/1 -> Delay7/1
  Delay3/1 -> Add/2
  LoD_3/1 -> Multiply/1
  Add3/1 -> Out_LoD_o/1
  Multiply/1 -> Add/1
  Multiply4/1 -> Add3/1
  Multiply1/1 -> Add1/1
  Delay6/1 -> Rate Transition2/1
  In_LoD_o/1 -> Delay1/1, Multiply4/2
  LoD_1/1 -> Multiply4/1
  Delay1/1 -> Rate Transition/1

== system final_heart_sym4_7_Level_double/3rd_Level_Recon/HiR_Even ==
  In_HiR_e : Inport  OutDataTypeStr=double  SampleTime=1/44100
  Add1 : Sum  AccumDataTypeStr=double  OutDataTypeStr=double
  Add2 : Sum  AccumDataTypeStr=double  OutDataTypeStr=double
  Add3 : Sum  AccumDataTypeStr=double  OutDataTypeStr=double
  Delay{1..3,5..7} (6 alike) : Delay  DelayLength=1  SampleTime=1/44100
  HiR_0 : Constant  Value=-0.075765715  OutDataTypeStr=double  SampleTime=1/44100
  HiR_2 : Constant  Value=0.497618668  OutDataTypeStr=double  SampleTime=1/44100
  HiR_4 : Constant  Value=0.297857796  OutDataTypeStr=double  SampleTime=1/44100
  HiR_6 : Constant  Value=-0.012603967  OutDataTypeStr=double  SampleTime=1/44100
  Multiply{1..4} (4 alike) : Product  OutDataTypeStr=double
  Rate Transition : RateTransition  OutPortSampleTime=1/44100
  Rate Transition1 : RateTransition  OutPortSampleTime=1/44100
  Rate Transition2 : RateTransition  OutPortSampleTime=1/44100
  Out_HiR_e : Outport  OutDataTypeStr=double  SampleTime=1/44100  VectorParamsAs1DForOutWhenUnconnected=off
  wires:
  In_HiR_e/1 -> Delay1/1, Multiply4/2
  Delay6/1 -> Rate Transition2/1
  Multiply2/1 -> Add2/1
  Rate Transition/1 -> Delay5/1, Multiply1/2
  HiR_6/1 -> Multiply3/1
  Multiply3/1 -> Delay2/1
  Delay2/1 -> Add2/2
  Rate Transition2/1 -> Multiply3/2
  Add3/1 -> Out_HiR_e/1
  Multiply1/1 -> Add1/1
  Delay1/1 -> Rate Transition/1
  Multiply4/1 -> Add3/1
  Add1/1 -> Delay7/1
  Add2/1 -> Delay3/1
  HiR_2/1 -> Multiply1/1
  HiR_4/1 -> Multiply2/1
  Delay7/1 -> Add3/2
  HiR_0/1 -> Multiply4/1
  Delay3/1 -> Add1/2
  Delay5/1 -> Rate Transition1/1
  Rate Transition1/1 -> Delay6/1, Multiply2/2

== system final_heart_sym4_7_Level_double/3rd_Level_Recon/HiR_Odd ==
  In_HiR_o : Inport  OutDataTypeStr=double  SampleTime=1/44100
  Add1 : Sum  AccumDataTypeStr=double  OutDataTypeStr=double
  Add2 : Sum  AccumDataTypeStr=double  OutDataTypeStr=double
  Add3 : Sum  AccumDataTypeStr=double  OutDataTypeStr=double
  Delay{1..3,5..7} (6 alike) : Delay  DelayLength=1  SampleTime=1/44100
  HiR_1 : Constant  Value=0.029635528  OutDataTypeStr=double  SampleTime=1/44100
  HiR_3 : Constant  Value=-0.803738752  OutDataTypeStr=double  SampleTime=1/44100
  HiR_5 : Constant  Value=0.099219544  OutDataTypeStr=double  SampleTime=1/44100
  HiR_7 : Constant  Value=-0.032223101  OutDataTypeStr=double  SampleTime=1/44100
  Multiply{1..4} (4 alike) : Product  OutDataTypeStr=double
  Rate Transition : RateTransition  OutPortSampleTime=1/44100
  Rate Transition1 : RateTransition  OutPortSampleTime=1/44100
  Rate Transition2 : RateTransition  OutPortSampleTime=1/44100
  Out_HiR_o : Outport  OutDataTypeStr=double  SampleTime=1/44100  VectorParamsAs1DForOutWhenUnconnected=off
  wires:
  Delay1/1 -> Rate Transition/1
  Multiply1/1 -> Add1/1
  Multiply3/1 -> Delay2/1
  Rate Transition2/1 -> Multiply3/2
  Delay2/1 -> Add2/2
  Rate Transition/1 -> Delay5/1, Multiply1/2
  Multiply2/1 -> Add2/1
  Add3/1 -> Out_HiR_o/1
  Delay6/1 -> Rate Transition2/1
  In_HiR_o/1 -> Delay1/1, Multiply4/2
  Delay7/1 -> Add3/2
  Multiply4/1 -> Add3/1
  HiR_3/1 -> Multiply1/1
  Add2/1 -> Delay3/1
  Delay5/1 -> Rate Transition1/1
  HiR_5/1 -> Multiply2/1
  Delay3/1 -> Add1/2
  Rate Transition1/1 -> Delay6/1, Multiply2/2
  Add1/1 -> Delay7/1
  HiR_1/1 -> Multiply4/1
  HiR_7/1 -> Multiply3/1

== system final_heart_sym4_7_Level_double/3rd_Level_Recon/LoR_Even ==
  In_LoR_e : Inport  OutDataTypeStr=double  SampleTime=1/44100
  Add1 : Sum  AccumDataTypeStr=double  OutDataTypeStr=double
  Add2 : Sum  AccumDataTypeStr=double  OutDataTypeStr=double
  Add3 : Sum  AccumDataTypeStr=double  OutDataTypeStr=double
  Delay{1..3,5..7} (6 alike) : Delay  DelayLength=1  SampleTime=1/44100
  LoR_0 : Constant  Value=0.032223101  OutDataTypeStr=double  SampleTime=1/44100
  LoR_2 : Constant  Value=-0.099219544  OutDataTypeStr=double  SampleTime=1/44100
  LoR_4 : Constant  Value=0.803738752  OutDataTypeStr=double  SampleTime=1/44100
  LoR_6 : Constant  Value=-0.029635528  OutDataTypeStr=double  SampleTime=1/44100
  Multiply{1..4} (4 alike) : Product  OutDataTypeStr=double
  Rate Transition : RateTransition  OutPortSampleTime=1/44100
  Rate Transition1 : RateTransition  OutPortSampleTime=1/44100
  Rate Transition2 : RateTransition  OutPortSampleTime=1/44100
  Out_LoR_e : Outport  OutDataTypeStr=double  SampleTime=1/44100  VectorParamsAs1DForOutWhenUnconnected=off
  wires:
  Delay1/1 -> Rate Transition/1
  Multiply1/1 -> Add1/1
  Multiply3/1 -> Delay2/1
  Rate Transition2/1 -> Multiply3/2
  Delay2/1 -> Add2/2
  Rate Transition/1 -> Delay5/1, Multiply1/2
  Multiply2/1 -> Add2/1
  Add3/1 -> Out_LoR_e/1
  Delay6/1 -> Rate Transition2/1
  In_LoR_e/1 -> Delay1/1, Multiply4/2
  Delay7/1 -> Add3/2
  Multiply4/1 -> Add3/1
  LoR_2/1 -> Multiply1/1
  Add2/1 -> Delay3/1
  Delay5/1 -> Rate Transition1/1
  LoR_4/1 -> Multiply2/1
  Delay3/1 -> Add1/2
  Rate Transition1/1 -> Delay6/1, Multiply2/2
  Add1/1 -> Delay7/1
  LoR_0/1 -> Multiply4/1
  LoR_6/1 -> Multiply3/1

== system final_heart_sym4_7_Level_double/3rd_Level_Recon/LoR_Odd ==
  In_LoR_o : Inport  OutDataTypeStr=double  SampleTime=1/44100
  Add1 : Sum  AccumDataTypeStr=double  OutDataTypeStr=double
  Add2 : Sum  AccumDataTypeStr=double  OutDataTypeStr=double
  Add3 : Sum  AccumDataTypeStr=double  OutDataTypeStr=double
  Delay{1..3,5..7} (6 alike) : Delay  DelayLength=1  SampleTime=1/44100
  LoR_1 : Constant  Value=-0.012603967  OutDataTypeStr=double  SampleTime=1/44100
  LoR_3 : Constant  Value=0.297857796  OutDataTypeStr=double  SampleTime=1/44100
  LoR_5 : Constant  Value=0.497618668  OutDataTypeStr=double  SampleTime=1/44100
  LoR_7 : Constant  Value=-0.075765715  OutDataTypeStr=double  SampleTime=1/44100
  Multiply{1..4} (4 alike) : Product  OutDataTypeStr=double
  Rate Transition : RateTransition  OutPortSampleTime=1/44100
  Rate Transition1 : RateTransition  OutPortSampleTime=1/44100
  Rate Transition2 : RateTransition  OutPortSampleTime=1/44100
  Out_LoR_o : Outport  OutDataTypeStr=double  SampleTime=1/44100  VectorParamsAs1DForOutWhenUnconnected=off
  wires:
  Rate Transition1/1 -> Delay6/1, Multiply2/2
  Add1/1 -> Delay7/1
  LoR_1/1 -> Multiply4/1
  LoR_7/1 -> Multiply3/1
  Delay3/1 -> Add1/2
  LoR_3/1 -> Multiply1/1
  Add2/1 -> Delay3/1
  LoR_5/1 -> Multiply2/1
  Delay5/1 -> Rate Transition1/1
  In_LoR_o/1 -> Delay1/1, Multiply4/2
  Multiply4/1 -> Add3/1
  Delay7/1 -> Add3/2
  Multiply2/1 -> Add2/1
  Rate Transition/1 -> Delay5/1, Multiply1/2
  Delay6/1 -> Rate Transition2/1
  Add3/1 -> Out_LoR_o/1
  Delay2/1 -> Add2/2
  Multiply3/1 -> Delay2/1
  Rate Transition2/1 -> Multiply3/2
  Multiply1/1 -> Add1/1
  Delay1/1 -> Rate Transition/1

== system final_heart_sym4_7_Level_double/4th_Level_Decomp/HiD_Even ==
  In_HiD_e : Inport  OutDataTypeStr=double  SampleTime=1/44100
  Add : Sum  AccumDataTypeStr=double  OutDataTypeStr=double
  Add1 : Sum  AccumDataTypeStr=double  OutDataTypeStr=double
  Add3 : Sum  AccumDataTypeStr=double  OutDataTypeStr=double
  Delay{1..3,5..7} (6 alike) : Delay  DelayLength=1  SampleTime=1/44100
  HiD_0 : Constant  Value=-0.032223101  OutDataTypeStr=double  SampleTime=1/44100
  HiD_2 : Constant  Value=0.099219544  OutDataTypeStr=double  SampleTime=1/44100
  HiD_4 : Constant  Value=-0.803738752  OutDataTypeStr=double  SampleTime=1/44100
  HiD_6 : Constant  Value=0.029635528  OutDataTypeStr=double  SampleTime=1/44100
  Multiply{,1..2,4} (4 alike) : Product  OutDataTypeStr=double
  Rate Transition : RateTransition  OutPortSampleTime=1/44100
  Rate Transition1 : RateTransition  OutPortSampleTime=1/44100
  Rate Transition2 : RateTransition  OutPortSampleTime=1/44100
  Out_HiD_e : Outport  OutDataTypeStr=double  SampleTime=1/44100  VectorParamsAs1DForOutWhenUnconnected=off
  wires:
  Rate Transition2/1 -> Multiply2/2
  Multiply2/1 -> Delay7/1
  HiD_0/1 -> Multiply4/1
  Delay3/1 -> Add/2
  HiD_6/1 -> Multiply2/1
  In_HiD_e/1 -> Delay1/1, Multiply4/2
  HiD_2/1 -> Multiply/1
  Add3/1 -> Out_HiD_e/1
  Multiply/1 -> Add/1
  Rate Transition/1 -> Delay5/1, Multiply/2
  HiD_4/1 -> Multiply1/1
  Delay6/1 -> Rate Transition2/1
  Delay1/1 -> Rate Transition/1
  Delay7/1 -> Add1/2
  Multiply1/1 -> Add1/1
  Rate Transition1/1 -> Delay6/1, Multiply1/2
  Delay2/1 -> Add3/2
  Multiply4/1 -> Add3/1
  Delay5/1 -> Rate Transition1/1
  Add/1 -> Delay2/1
  Add1/1 -> Delay3/1

== system final_heart_sym4_7_Level_double/4th_Level_Decomp/HiD_Odd ==
  In_HiD_o : Inport  OutDataTypeStr=double  SampleTime=1/44100
  Add : Sum  AccumDataTypeStr=double  OutDataTypeStr=double
  Add1 : Sum  AccumDataTypeStr=double  OutDataTypeStr=double
  Add3 : Sum  AccumDataTypeStr=double  OutDataTypeStr=double
  Delay{1..3,5..7} (6 alike) : Delay  DelayLength=1  SampleTime=1/44100
  HiD_1 : Constant  Value=-0.012603967  OutDataTypeStr=double  SampleTime=1/44100
  HiD_3 : Constant  Value=0.297857796  OutDataTypeStr=double  SampleTime=1/44100
  HiD_5 : Constant  Value=0.497618668  OutDataTypeStr=double  SampleTime=1/44100
  HiD_7 : Constant  Value=-0.075765715  OutDataTypeStr=double  SampleTime=1/44100
  Multiply{,1..2,4} (4 alike) : Product  OutDataTypeStr=double
  Rate Transition : RateTransition  OutPortSampleTime=1/44100
  Rate Transition1 : RateTransition  OutPortSampleTime=1/44100
  Rate Transition2 : RateTransition  OutPortSampleTime=1/44100
  Out_HiD_o : Outport  OutDataTypeStr=double  SampleTime=1/44100  VectorParamsAs1DForOutWhenUnconnected=off
  wires:
  Delay1/1 -> Rate Transition/1
  Delay6/1 -> Rate Transition2/1
  Rate Transition/1 -> Delay5/1, Multiply/2
  HiD_5/1 -> Multiply1/1
  Rate Transition1/1 -> Delay6/1, Multiply1/2
  Delay2/1 -> Add3/2
  Multiply1/1 -> Add1/1
  Add1/1 -> Delay3/1
  Delay5/1 -> Rate Transition1/1
  Delay7/1 -> Add1/2
  Add/1 -> Delay2/1
  In_HiD_o/1 -> Delay1/1, Multiply4/2
  Multiply4/1 -> Add3/1
  Multiply/1 -> Add/1
  Add3/1 -> Out_HiD_o/1
  HiD_3/1 -> Multiply/1
  HiD_1/1 -> Multiply4/1
  Delay3/1 -> Add/2
  Multiply2/1 -> Delay7/1
  Rate Transition2/1 -> Multiply2/2
  HiD_7/1 -> Multiply2/1

== system final_heart_sym4_7_Level_double/4th_Level_Decomp/LoD_Even ==
  In_LoD_e : Inport  OutDataTypeStr=double  SampleTime=1/44100
  Add : Sum  AccumDataTypeStr=double  OutDataTypeStr=double
  Add1 : Sum  AccumDataTypeStr=double  OutDataTypeStr=double
  Add3 : Sum  AccumDataTypeStr=double  OutDataTypeStr=double
  Delay{1..3,5..7} (6 alike) : Delay  DelayLength=1  SampleTime=1/44100
  LoD_0 : Constant  Value=-0.075765715  OutDataTypeStr=double  SampleTime=1/44100
  LoD_2 : Constant  Value=0.497618668  OutDataTypeStr=double  SampleTime=1/44100
  LoD_4 : Constant  Value=0.297857796  OutDataTypeStr=double  SampleTime=1/44100
  LoD_6 : Constant  Value=-0.012603967  OutDataTypeStr=double  SampleTime=1/44100
  Multiply{,1..2,4} (4 alike) : Product  OutDataTypeStr=double
  Rate Transition : RateTransition  OutPortSampleTime=1/44100
  Rate Transition1 : RateTransition  OutPortSampleTime=1/44100
  Rate Transition2 : RateTransition  OutPortSampleTime=1/44100
  Out_LoD_e : Outport  OutDataTypeStr=double  SampleTime=1/44100  VectorParamsAs1DForOutWhenUnconnected=off
  wires:
  Delay1/1 -> Rate Transition/1
  Delay6/1 -> Rate Transition2/1
  Rate Transition/1 -> Delay5/1, Multiply/2
  LoD_4/1 -> Multiply1/1
  Rate Transition1/1 -> Delay6/1, Multiply1/2
  Delay2/1 -> Add3/2
  Multiply1/1 -> Add1/1
  Add1/1 -> Delay3/1
  Delay5/1 -> Rate Transition1/1
  Delay7/1 -> Add1/2
  Add/1 -> Delay2/1
  In_LoD_e/1 -> Delay1/1, Multiply4/2
  Multiply4/1 -> Add3/1
  Multiply/1 -> Add/1
  Add3/1 -> Out_LoD_e/1
  LoD_2/1 -> Multiply/1
  LoD_0/1 -> Multiply4/1
  Delay3/1 -> Add/2
  Multiply2/1 -> Delay7/1
  Rate Transition2/1 -> Multiply2/2
  LoD_6/1 -> Multiply2/1

== system final_heart_sym4_7_Level_double/4th_Level_Decomp/LoD_Odd ==
  In_LoD_o : Inport  OutDataTypeStr=double  SampleTime=1/44100
  Add : Sum  AccumDataTypeStr=double  OutDataTypeStr=double
  Add1 : Sum  AccumDataTypeStr=double  OutDataTypeStr=double
  Add3 : Sum  AccumDataTypeStr=double  OutDataTypeStr=double
  Delay{1..3,5..7} (6 alike) : Delay  DelayLength=1  SampleTime=1/44100
  LoD_1 : Constant  Value=-0.029635528  OutDataTypeStr=double  SampleTime=1/44100
  LoD_3 : Constant  Value=0.803738752  OutDataTypeStr=double  SampleTime=1/44100
  LoD_5 : Constant  Value=-0.099219544  OutDataTypeStr=double  SampleTime=1/44100
  LoD_7 : Constant  Value=0.032223101  OutDataTypeStr=double  SampleTime=1/44100
  Multiply{,1..2,4} (4 alike) : Product  OutDataTypeStr=double
  Rate Transition : RateTransition  OutPortSampleTime=1/44100
  Rate Transition1 : RateTransition  OutPortSampleTime=1/44100
  Rate Transition2 : RateTransition  OutPortSampleTime=1/44100
  Out_LoD_o : Outport  OutDataTypeStr=double  SampleTime=1/44100  VectorParamsAs1DForOutWhenUnconnected=off
  wires:
  Rate Transition/1 -> Delay5/1, Multiply/2
  Add/1 -> Delay2/1
  Add1/1 -> Delay3/1
  Delay7/1 -> Add1/2
  Delay5/1 -> Rate Transition1/1
  Rate Transition1/1 -> Delay6/1, Multiply1/2
  Delay2/1 -> Add3/2
  LoD_5/1 -> Multiply1/1
  Rate Transition2/1 -> Multiply2/2
  LoD_7/1 -> Multiply2/1
  Multiply2/1 -> Delay7/1
  Delay3/1 -> Add/2
  LoD_3/1 -> Multiply/1
  Add3/1 -> Out_LoD_o/1
  Multiply/1 -> Add/1
  Multiply4/1 -> Add3/1
  Multiply1/1 -> Add1/1
  Delay6/1 -> Rate Transition2/1
  In_LoD_o/1 -> Delay1/1, Multiply4/2
  LoD_1/1 -> Multiply4/1
  Delay1/1 -> Rate Transition/1

== system final_heart_sym4_7_Level_double/4th_Level_Recon/HiR_Even ==
  In_HiR_e : Inport  OutDataTypeStr=double  SampleTime=1/44100
  Add1 : Sum  AccumDataTypeStr=double  OutDataTypeStr=double
  Add2 : Sum  AccumDataTypeStr=double  OutDataTypeStr=double
  Add3 : Sum  AccumDataTypeStr=double  OutDataTypeStr=double
  Delay{1..3,5..7} (6 alike) : Delay  DelayLength=1  SampleTime=1/44100
  HiR_0 : Constant  Value=-0.075765715  OutDataTypeStr=double  SampleTime=1/44100
  HiR_2 : Constant  Value=0.497618668  OutDataTypeStr=double  SampleTime=1/44100
  HiR_4 : Constant  Value=0.297857796  OutDataTypeStr=double  SampleTime=1/44100
  HiR_6 : Constant  Value=-0.012603967  OutDataTypeStr=double  SampleTime=1/44100
  Multiply{1..4} (4 alike) : Product  OutDataTypeStr=double
  Rate Transition : RateTransition  OutPortSampleTime=1/44100
  Rate Transition1 : RateTransition  OutPortSampleTime=1/44100
  Rate Transition2 : RateTransition  OutPortSampleTime=1/44100
  Out_HiR_e : Outport  OutDataTypeStr=double  SampleTime=1/44100  VectorParamsAs1DForOutWhenUnconnected=off
  wires:
  In_HiR_e/1 -> Delay1/1, Multiply4/2
  Delay6/1 -> Rate Transition2/1
  Multiply2/1 -> Add2/1
  Rate Transition/1 -> Delay5/1, Multiply1/2
  HiR_6/1 -> Multiply3/1
  Multiply3/1 -> Delay2/1
  Delay2/1 -> Add2/2
  Rate Transition2/1 -> Multiply3/2
  Add3/1 -> Out_HiR_e/1
  Multiply1/1 -> Add1/1
  Delay1/1 -> Rate Transition/1
  Multiply4/1 -> Add3/1
  Add1/1 -> Delay7/1
  Add2/1 -> Delay3/1
  HiR_2/1 -> Multiply1/1
  HiR_4/1 -> Multiply2/1
  Delay7/1 -> Add3/2
  HiR_0/1 -> Multiply4/1
  Delay3/1 -> Add1/2
  Delay5/1 -> Rate Transition1/1
  Rate Transition1/1 -> Delay6/1, Multiply2/2
